simulink model "parallel_downconverter_test"  (Simulink 7.4)
settings: Solver=ode45  StartTime=0.0  StopTime=1000  RelTol=1e-3
undefined symbols (not defined in the file): Parallel_scope, Parallelizer, To_be_added_to_xBlocks_devels
libraries: xbsIndex_r4 x73, simulink x5
settings Model: Creator=chenhong  LastModifiedBy=hong

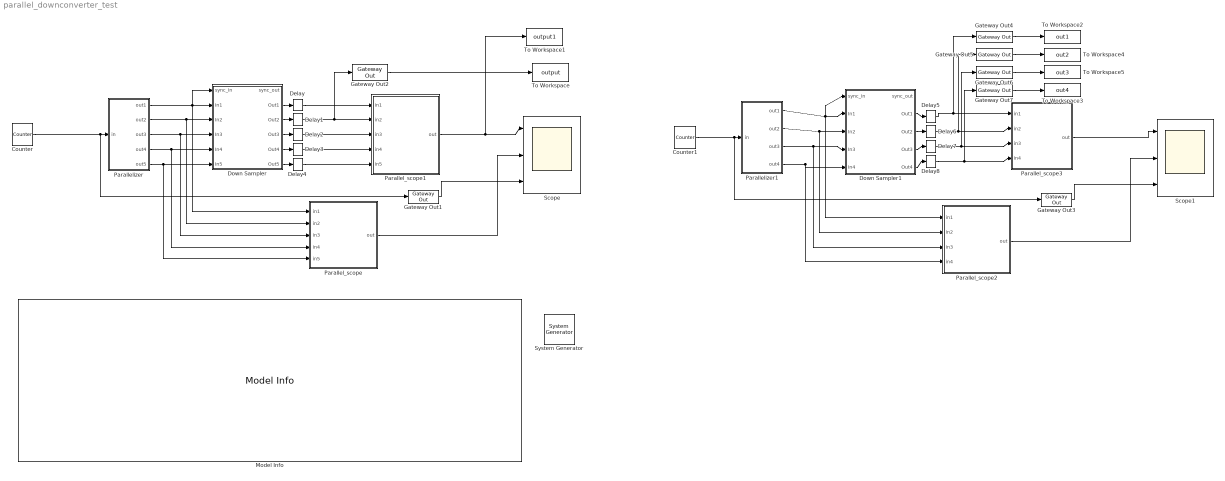
== system parallel_downconverter_test ==
  " System Generator" : xbsIndex_r4/ System Generator  Tag=genX  SystemSampleTime=-1  xilinxfamily=virtex6  part=xc6vsx315t  speed=-3  package=ff1156  synthesis_tool=XST  clock_wrapper=Clock Enables  directory=./netlist  testbench=off  simulink_period=1  sysclk_period=10  dcm_input_clock_period=10  incr_netlist=off  trim_vbits=Everywhere in SubSystem  dbl_ovrd=According to Block Masks  core_generation=According to Block Masks  run_coregen=off  deprecated_control=off  eval_field=0  block_type=sysgen
      settings: block_version=11.4
  Counter : xbsIndex_r4/Counter  cnt_type=Free Running  cnt_to=Inf  operation=Up  start_count=0  cnt_by_val=1  arith_type=Unsigned  n_bits=8  bin_pt=0  load_pin=off  rst=off  en=off  explicit_period=on  period=1  dbl_ovrd=off  use_behavioral_HDL=off  implementation=Fabric  block_type=counter
      settings: block_version=11.4
  Counter1 : xbsIndex_r4/Counter  cnt_type=Free Running  cnt_to=Inf  operation=Up  start_count=0  cnt_by_val=1  arith_type=Unsigned  n_bits=8  bin_pt=0  load_pin=off  rst=off  en=off  explicit_period=on  period=1  dbl_ovrd=off  use_behavioral_HDL=off  implementation=Fabric  block_type=counter
      settings: block_version=11.4
  Delay{,1..8} (9 alike) : xbsIndex_r4/Delay  en=off  latency=7  dbl_ovrd=off  reg_retiming=off  block_type=delay
      settings: block_version=11.4
  Down Sampler : Subsystem  mask(Parallel Downconverter (xBlock)){n_inputs=5, dec_rate=2, xilinx=off, input_clk_rate=5}
      mask prompts: n_inputs "number of inputs"; dec_rate "Decimation rate"; xilinx "Use Xilinx version of Down Sample?"; input_clk_rate "Input Clock Rate"
      mask help: Parallely downconvert.
      mask init:
      | config.source=str2func('parallel_downsampler_init_xblock');
      | config.depend=get_dependlist('parallel_downsampler');
      | config.toplevel=gcb;
      | set_param(gcb,'LinkStatus','inactive');
      | xBlock(config, {config.toplevel,...
      |     'n_inputs', n_inputs, ...
      |     'dec_rate', dec_rate, ...
      |     'xilinx', xilinx, ...
      |     'input_clk_rate', input_clk_rate});
      settings: AttributesFormatString=Decimation Rate = 2
  Down Sampler1 : Subsystem  mask(Parallel Downconverter (xBlock)){n_inputs=4, dec_rate=2, xilinx=off, input_clk_rate=4}
      mask prompts: n_inputs "number of inputs"; dec_rate "Decimation rate"; xilinx "Use Xilinx version of Down Sample?"; input_clk_rate "Input Clock Rate"
      mask help: Parallely downconvert.
      mask init: same as parallel_downconverter_test/Down Sampler
      settings: AttributesFormatString=Decimation Rate = 2
  Gateway Out{1..7} (7 alike) : xbsIndex_r4/Gateway Out  hdl_port=on  timing_constraint=None  locs_specified=off  LOCs={}  block_type=gatewayout
      settings: infoedit="Gateway out block.  Converts Xilinx fixed point inputs into ouputs of type Simulink integer, double, or fixed point.<br><br>Hardware notes:  In hardware these blocks become top level output ports or are discarded, depending on how they are configured."  block_version=11.4
  Model Info : simulink/Model-Wide Utilities/Model Info  SystemSampleTime=-1  InitialBlockCM=None  BlockCM=None  Frame=on  DisplayStringWithTags=|  HorizontalTextAlignment=Center  LeftAlignmentValue=0.5  SourceBlockDiagram=parallel_downconverter_test  TagMaxNumber=20
      | January 18, 2012:
      | 
      | Test passed.
      | 
      | Used downsample_init_xblock instead of the xilinx Down Sample block. Note that in this case it doesn't really change the sampling rate, just hold a certain value for a specific time. Therefore we need to adjust delays to see how they're matched.
      | 
      | To do: add option to choose the first value or last value in a single time frame.
      | 
      | 
      | ---------------------------------------------------------------
      | September 28, 2011:
      | 
      | Test passed. 
      | 
      | The counter generates 1-D discrete samples at 1 sample/clk rate. The parallelizer outputs 4-parallel outputs
      | at 4 sample/clk. The downconverter downsample to 4/dec_rate sample/clk. After the serializer, the final 1-D output stream is 1/dec_rate sample/clk.
      | 
      | 
      | Also tested: 5-parallel inputs; various dec_rate
  Parallel_scope : Subsystem  AncestorBlock=To_be_added_to_xBlocks_devels/Parallel_scope  mask(Parallel Scope){n_inputs=5, sample_period=5}
      mask prompts: n_inputs "Number of inputs"; sample_period "Sample Period"
      mask help:
      | This parallel scope can handle parallel inputs
      | by propagating though gateways and serialize into
      | one single stream. The output can then be connected
      | directly to a scope or toWorkspace.
      |
      | The sample_period desribes the parallel inputs rate.
      | For example, for a 4-inputs stream with sample_period = 1
      | (4 parallel inputs per Clk),  the output stream frequency
      | would be 4/1 = 4 (Sample/Clk)
      mask init:
      | config.source=str2func('parallel_scope_init_xblock');
      | config.depend=get_dependlist('parallel_scope');
      | config.toplevel=gcb;
      | set_param(gcb,'LinkStatus','inactive');
      | xBlock(config, {config.toplevel,...
      |     'n_inputs', n_inputs, ...
      |     'sample_period', sample_period});
      settings: AttributesFormatString=Sample Period = 5
  Parallel_scope1 : Subsystem  mask(Parallel Scope){n_inputs=5, sample_period=10, explicit_period=off}
      mask prompts: n_inputs "Number of inputs"; sample_period "Sample Period"; explicit_period "Explicit Period?"
      mask help:
      | This parallel scope can handle parallel inputs
      | by propagating though gateways and serialize into
      | one single stream. The output can then be connected
      | directly to a scope or toWorkspace.
      |
      | The sample_period desribes the parallel inputs rate.
      | For example, for a 4-inputs stream with sample_period = 1
      | (4 parallel inputs per Clk),  the output stream frequency
      | would be 4/1 = 4 (Sample/Clk)
      mask init:
      | config.source=str2func('parallel_scope_init_xblock');
      | config.depend=get_dependlist('parallel_scope');
      | config.toplevel=gcb;
      | set_param(gcb,'LinkStatus','inactive');
      | xBlock(config, {config.toplevel,...
      |     'n_inputs', n_inputs, ...
      |     'sample_period', sample_period, ...
      |     'explicit_period', explicit_period});
      settings: AttributesFormatString=Sample Period = 10
  Parallel_scope2 : Subsystem  AncestorBlock=To_be_added_to_xBlocks_devels/Parallel_scope  mask(Parallel Scope){n_inputs=4, sample_period=4}
      mask prompts: n_inputs "Number of inputs"; sample_period "Sample Period"
      mask help:
      | This parallel scope can handle parallel inputs
      | by propagating though gateways and serialize into
      | one single stream. The output can then be connected
      | directly to a scope or toWorkspace.
      |
      | The sample_period desribes the parallel inputs rate.
      | For example, for a 4-inputs stream with sample_period = 1
      | (4 parallel inputs per Clk),  the output stream frequency
      | would be 4/1 = 4 (Sample/Clk)
      mask init: same as parallel_downconverter_test/Parallel_scope
      settings: AttributesFormatString=Sample Period = 4
  Parallel_scope3 : Subsystem  mask(Parallel Scope){n_inputs=4, sample_period=8, explicit_period=off}
      mask prompts: n_inputs "Number of inputs"; sample_period "Sample Period"; explicit_period "Explicit Period?"
      mask help:
      | This parallel scope can handle parallel inputs
      | by propagating though gateways and serialize into
      | one single stream. The output can then be connected
      | directly to a scope or toWorkspace.
      |
      | The sample_period desribes the parallel inputs rate.
      | For example, for a 4-inputs stream with sample_period = 1
      | (4 parallel inputs per Clk),  the output stream frequency
      | would be 4/1 = 4 (Sample/Clk)
      mask init: same as parallel_downconverter_test/Parallel_scope1
      settings: AttributesFormatString=Sample Period = 8
  Parallelizer : Subsystem  AncestorBlock=To_be_added_to_xBlocks_devels/Parallelizer  mask(Parallelizer){n_outputs=5, sample_period=1}
      mask help:
      | Parallelizer takes in a single stream and convert it into
      | parallel outputs
      mask init:
      | config.source=str2func('parallelizer_init_xblock');
      | config.depend=get_dependlist('parallelizer');
      | config.toplevel=gcb;
      | set_param(gcb,'LinkStatus','inactive');
      | xBlock(config, {config.toplevel,...
      |     'n_outputs', n_outputs, ...
      |     'sample_period', sample_period});
      settings: AttributesFormatString=Sample Period = 1
  Parallelizer1 : Subsystem  AncestorBlock=To_be_added_to_xBlocks_devels/Parallelizer  mask(Parallelizer){n_outputs=4, sample_period=1}
      mask help:
      | Parallelizer takes in a single stream and convert it into
      | parallel outputs
      mask init: same as parallel_downconverter_test/Parallelizer
      settings: AttributesFormatString=Sample Period = 1
  Scope : Scope  NumInputPorts=3
      settings: YMin=-5~-5~-5  YMax=5~5~5
  Scope1 : Scope  NumInputPorts=3
      settings: YMin=-5~-5~-5  YMax=5~5~5
  To Workspace : ToWorkspace  VariableName=output  SampleTime=-1  SaveFormat=Structure
  To Workspace1 : ToWorkspace  VariableName=output1  SampleTime=-1  SaveFormat=Structure
  To Workspace2 : ToWorkspace  VariableName=out1  SampleTime=-1  SaveFormat=Structure
  To Workspace3 : ToWorkspace  VariableName=out4  SampleTime=-1  SaveFormat=Structure
  To Workspace4 : ToWorkspace  VariableName=out2  SampleTime=-1  SaveFormat=Structure
  To Workspace5 : ToWorkspace  VariableName=out3  SampleTime=-1  SaveFormat=Structure
  wires:
  Counter/1 -> Parallelizer/1(in), Gateway Out1/1
  Parallelizer/1(out1) -> Parallel_scope/1(in1), Down Sampler/1(sync_in), Down Sampler/2(In1)
  Parallelizer/2(out2) -> Parallel_scope/2(in2), Down Sampler/3(In2)
  Parallelizer/3(out3) -> Parallel_scope/3(in3), Down Sampler/4(In3)
  Parallelizer/4(out4) -> Parallel_scope/4(in4), Down Sampler/5(In4)
  Down Sampler/2(Out1) -> Delay/1
  Down Sampler/3(Out2) -> Delay1/1
  Down Sampler/4(Out3) -> Delay2/1
  Down Sampler/5(Out4) -> Delay3/1
  Parallel_scope1/1(out) -> Scope/1, To Workspace1/1
  Parallel_scope/1(out) -> Scope/2
  Gateway Out1/1 -> Scope/3
  Parallelizer/5(out5) -> Parallel_scope/5(in5), Down Sampler/6(In5)
  Down Sampler/6(Out5) -> Delay4/1
  Gateway Out2/1 -> To Workspace/1
  Delay/1 -> Parallel_scope1/1(in1)
  Delay1/1 -> Parallel_scope1/2(in2), Gateway Out2/1
  Delay2/1 -> Parallel_scope1/3(in3)
  Delay3/1 -> Parallel_scope1/4(in4)
  Delay4/1 -> Parallel_scope1/5(in5)
  Counter1/1 -> Parallelizer1/1(in), Gateway Out3/1
  Parallelizer1/1(out1) -> Parallel_scope2/1(in1), Down Sampler1/1(sync_in), Down Sampler1/2(In1)
  Parallelizer1/2(out2) -> Parallel_scope2/2(in2), Down Sampler1/3(In2)
  Parallelizer1/3(out3) -> Parallel_scope2/3(in3), Down Sampler1/4(In3)
  Parallelizer1/4(out4) -> Parallel_scope2/4(in4), Down Sampler1/5(In4)
  Down Sampler1/2(Out1) -> Delay5/1
  Down Sampler1/3(Out2) -> Delay6/1
  Down Sampler1/4(Out3) -> Delay7/1
  Down Sampler1/5(Out4) -> Delay8/1
  Parallel_scope3/1(out) -> Scope1/1
  Parallel_scope2/1(out) -> Scope1/2
  Gateway Out3/1 -> Scope1/3
  Delay5/1 -> Parallel_scope3/1(in1), Gateway Out4/1
  Delay6/1 -> Parallel_scope3/2(in2), Gateway Out5/1
  Delay7/1 -> Parallel_scope3/3(in3), Gateway Out6/1
  Delay8/1 -> Parallel_scope3/4(in4), Gateway Out7/1
  Gateway Out4/1 -> To Workspace2/1
  Gateway Out5/1 -> To Workspace4/1
  Gateway Out6/1 -> To Workspace5/1
  Gateway Out7/1 -> To Workspace3/1

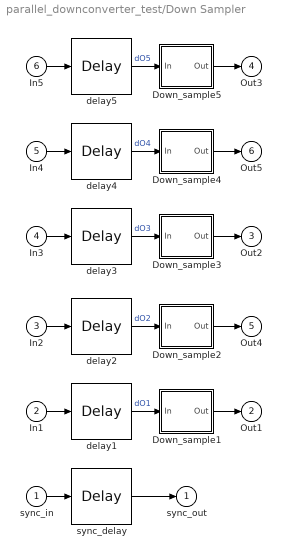
== system parallel_downconverter_test/Down Sampler ==
  sync_in : Inport
  In1 : Inport  Port=2
  In2 : Inport  Port=3
  In3 : Inport  Port=4
  In4 : Inport  Port=5
  In5 : Inport  Port=6
  Down_sample1 : Subsystem
  Down_sample2 : Subsystem
  Down_sample3 : Subsystem
  Down_sample4 : Subsystem
  Down_sample5 : Subsystem
  delay1 : xbsIndex_r4/Delay  en=off  latency=1  dbl_ovrd=off  reg_retiming=off  block_type=delay
      settings: block_version=11.4
  delay2 : xbsIndex_r4/Delay  en=off  latency=0  dbl_ovrd=off  reg_retiming=off  block_type=delay
      settings: block_version=11.4
  delay3 : xbsIndex_r4/Delay  en=off  latency=1  dbl_ovrd=off  reg_retiming=off  block_type=delay
      settings: block_version=11.4
  delay4 : xbsIndex_r4/Delay  en=off  latency=0  dbl_ovrd=off  reg_retiming=off  block_type=delay
      settings: block_version=11.4
  delay5 : xbsIndex_r4/Delay  en=off  latency=1  dbl_ovrd=off  reg_retiming=off  block_type=delay
      settings: block_version=11.4
  sync_delay : xbsIndex_r4/Delay  en=off  latency=1  dbl_ovrd=off  reg_retiming=off  block_type=delay
      settings: block_version=11.4
  sync_out : Outport
  Out1 : Outport  Port=2
  Out2 : Outport  Port=3
  Out3 : Outport  Port=4
  Out4 : Outport  Port=5
  Out5 : Outport  Port=6
  wires:
  sync_delay/1 -> sync_out/1
  sync_in/1 -> sync_delay/1
  Down_sample5/1(Out) -> Out3/1
  delay5/1 -> Down_sample5/1(In)  "dO5"
  In5/1 -> delay5/1
  Down_sample4/1(Out) -> Out5/1
  delay4/1 -> Down_sample4/1(In)  "dO4"
  In4/1 -> delay4/1
  Down_sample3/1(Out) -> Out2/1
  delay3/1 -> Down_sample3/1(In)  "dO3"
  In3/1 -> delay3/1
  Down_sample2/1(Out) -> Out4/1
  delay2/1 -> Down_sample2/1(In)  "dO2"
  In2/1 -> delay2/1
  Down_sample1/1(Out) -> Out1/1
  delay1/1 -> Down_sample1/1(In)  "dO1"
  In1/1 -> delay1/1

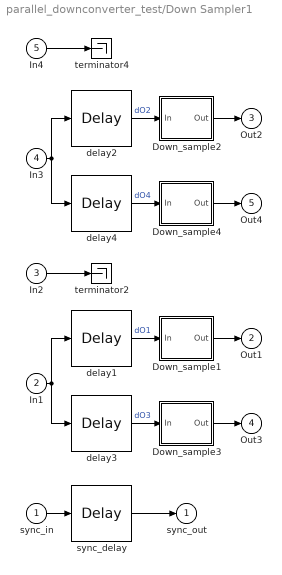
== system parallel_downconverter_test/Down Sampler1 ==
  sync_in : Inport
  In1 : Inport  Port=2
  In2 : Inport  Port=3
  In3 : Inport  Port=4
  In4 : Inport  Port=5
  Down_sample1 : Subsystem
  Down_sample2 : Subsystem
  Down_sample3 : Subsystem
  Down_sample4 : Subsystem
  delay1 : xbsIndex_r4/Delay  en=off  latency=1  dbl_ovrd=off  reg_retiming=off  block_type=delay
      settings: block_version=11.4
  delay2 : xbsIndex_r4/Delay  en=off  latency=1  dbl_ovrd=off  reg_retiming=off  block_type=delay
      settings: block_version=11.4
  delay3 : xbsIndex_r4/Delay  en=off  latency=0  dbl_ovrd=off  reg_retiming=off  block_type=delay
      settings: block_version=11.4
  delay4 : xbsIndex_r4/Delay  en=off  latency=0  dbl_ovrd=off  reg_retiming=off  block_type=delay
      settings: block_version=11.4
  sync_delay : xbsIndex_r4/Delay  en=off  latency=1  dbl_ovrd=off  reg_retiming=off  block_type=delay
      settings: block_version=11.4
  terminator2 : Terminator
  terminator4 : Terminator
  sync_out : Outport
  Out1 : Outport  Port=2
  Out2 : Outport  Port=3
  Out3 : Outport  Port=4
  Out4 : Outport  Port=5
  wires:
  In1/1 -> delay3/1, delay1/1
  In3/1 -> delay4/1, delay2/1
  sync_delay/1 -> sync_out/1
  sync_in/1 -> sync_delay/1
  Down_sample4/1(Out) -> Out4/1
  delay4/1 -> Down_sample4/1(In)  "dO4"
  Down_sample3/1(Out) -> Out3/1
  delay3/1 -> Down_sample3/1(In)  "dO3"
  Down_sample2/1(Out) -> Out2/1
  delay2/1 -> Down_sample2/1(In)  "dO2"
  Down_sample1/1(Out) -> Out1/1
  delay1/1 -> Down_sample1/1(In)  "dO1"
  In4/1 -> terminator4/1
  In2/1 -> terminator2/1

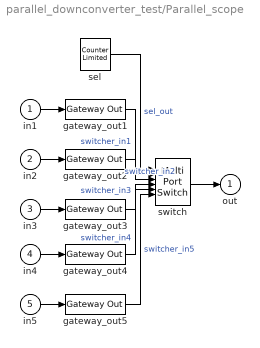
== system parallel_downconverter_test/Parallel_scope ==
  in1 : Inport
  in2 : Inport  Port=2
  in3 : Inport  Port=3
  in4 : Inport  Port=4
  in5 : Inport  Port=5
  gateway_out{1..5} (5 alike) : xbsIndex_r4/Gateway Out  hdl_port=off  timing_constraint=None  locs_specified=off  LOCs={}  block_type=gatewayout
      settings: infoedit="Gateway out block.  Converts Xilinx fixed point inputs into ouputs of type Simulink integer, double, or fixed point.<br><br>Hardware notes:  In hardware these blocks become top level output ports or are discarded, depending on how they are configured."  block_version=11.4
  sel : simulink/Sources/Counter Limited  SystemSampleTime=-1  uplimit=4  tsamp=1
  switch : MultiPortSwitch  Inputs=5  zeroidx=on  OutDataType=fixdt(1, 16)  OutScaling=2^0
  out : Outport
  wires:
  switch/1 -> out/1
  gateway_out5/1 -> switch/6  "switcher_in5"
  gateway_out4/1 -> switch/5  "switcher_in4"
  gateway_out3/1 -> switch/4  "switcher_in3"
  gateway_out2/1 -> switch/3  "switcher_in2"
  gateway_out1/1 -> switch/2  "switcher_in1"
  sel/1 -> switch/1  "sel_out"
  in5/1 -> gateway_out5/1
  in4/1 -> gateway_out4/1
  in3/1 -> gateway_out3/1
  in2/1 -> gateway_out2/1
  in1/1 -> gateway_out1/1

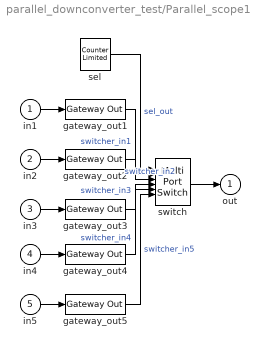
== system parallel_downconverter_test/Parallel_scope1 ==
  in1 : Inport
  in2 : Inport  Port=2
  in3 : Inport  Port=3
  in4 : Inport  Port=4
  in5 : Inport  Port=5
  gateway_out{1..5} (5 alike) : xbsIndex_r4/Gateway Out  hdl_port=off  timing_constraint=None  locs_specified=off  LOCs={}  block_type=gatewayout
      settings: infoedit="Gateway out block.  Converts Xilinx fixed point inputs into ouputs of type Simulink integer, double, or fixed point.<br><br>Hardware notes:  In hardware these blocks become top level output ports or are discarded, depending on how they are configured."  block_version=11.4
  sel : simulink/Sources/Counter Limited  SystemSampleTime=-1  uplimit=4  tsamp=2
  switch : MultiPortSwitch  Inputs=5  zeroidx=on  OutDataType=fixdt(1, 16)  OutScaling=2^0
  out : Outport
  wires:
  switch/1 -> out/1
  gateway_out5/1 -> switch/6  "switcher_in5"
  gateway_out4/1 -> switch/5  "switcher_in4"
  gateway_out3/1 -> switch/4  "switcher_in3"
  gateway_out2/1 -> switch/3  "switcher_in2"
  gateway_out1/1 -> switch/2  "switcher_in1"
  sel/1 -> switch/1  "sel_out"
  in5/1 -> gateway_out5/1
  in4/1 -> gateway_out4/1
  in3/1 -> gateway_out3/1
  in2/1 -> gateway_out2/1
  in1/1 -> gateway_out1/1

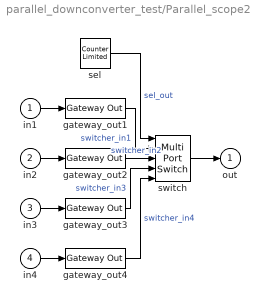
== system parallel_downconverter_test/Parallel_scope2 ==
  in1 : Inport
  in2 : Inport  Port=2
  in3 : Inport  Port=3
  in4 : Inport  Port=4
  gateway_out{1..4} (4 alike) : xbsIndex_r4/Gateway Out  hdl_port=off  timing_constraint=None  locs_specified=off  LOCs={}  block_type=gatewayout
      settings: infoedit="Gateway out block.  Converts Xilinx fixed point inputs into ouputs of type Simulink integer, double, or fixed point.<br><br>Hardware notes:  In hardware these blocks become top level output ports or are discarded, depending on how they are configured."  block_version=11.4
  sel : simulink/Sources/Counter Limited  SystemSampleTime=-1  uplimit=3  tsamp=1
  switch : MultiPortSwitch  Inputs=4  zeroidx=on  OutDataType=fixdt(1, 16)  OutScaling=2^0
  out : Outport
  wires:
  switch/1 -> out/1
  gateway_out4/1 -> switch/5  "switcher_in4"
  gateway_out3/1 -> switch/4  "switcher_in3"
  gateway_out2/1 -> switch/3  "switcher_in2"
  gateway_out1/1 -> switch/2  "switcher_in1"
  sel/1 -> switch/1  "sel_out"
  in4/1 -> gateway_out4/1
  in3/1 -> gateway_out3/1
  in2/1 -> gateway_out2/1
  in1/1 -> gateway_out1/1

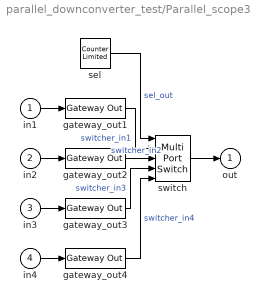
== system parallel_downconverter_test/Parallel_scope3 ==
  in1 : Inport
  in2 : Inport  Port=2
  in3 : Inport  Port=3
  in4 : Inport  Port=4
  gateway_out{1..4} (4 alike) : xbsIndex_r4/Gateway Out  hdl_port=off  timing_constraint=None  locs_specified=off  LOCs={}  block_type=gatewayout
      settings: infoedit="Gateway out block.  Converts Xilinx fixed point inputs into ouputs of type Simulink integer, double, or fixed point.<br><br>Hardware notes:  In hardware these blocks become top level output ports or are discarded, depending on how they are configured."  block_version=11.4
  sel : simulink/Sources/Counter Limited  SystemSampleTime=-1  uplimit=3  tsamp=2
  switch : MultiPortSwitch  Inputs=4  zeroidx=on  OutDataType=fixdt(1, 16)  OutScaling=2^0
  out : Outport
  wires:
  switch/1 -> out/1
  gateway_out4/1 -> switch/5  "switcher_in4"
  gateway_out3/1 -> switch/4  "switcher_in3"
  gateway_out2/1 -> switch/3  "switcher_in2"
  gateway_out1/1 -> switch/2  "switcher_in1"
  sel/1 -> switch/1  "sel_out"
  in4/1 -> gateway_out4/1
  in3/1 -> gateway_out3/1
  in2/1 -> gateway_out2/1
  in1/1 -> gateway_out1/1

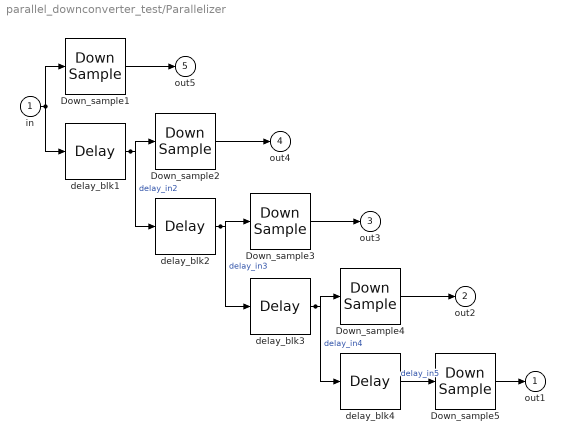
== system parallel_downconverter_test/Parallelizer ==
  in : Inport
  Down_sample{1..5} (5 alike) : xbsIndex_r4/Down Sample  sample_ratio=5  sample_phase="Last Value of Frame  (most efficient)"  en=off  latency=1  dbl_ovrd=off  block_type=dsamp
      settings: block_version=11.4
  delay_blk{1..4} (4 alike) : xbsIndex_r4/Delay  en=off  latency=1  dbl_ovrd=off  reg_retiming=off  block_type=delay
      settings: block_version=11.4
  out1 : Outport
  out2 : Outport  Port=2
  out3 : Outport  Port=3
  out4 : Outport  Port=4
  out5 : Outport  Port=5
  wires:
  in/1 -> Down_sample1/1, delay_blk1/1
  delay_blk1/1 -> Down_sample2/1, delay_blk2/1  "delay_in2"
  delay_blk2/1 -> Down_sample3/1, delay_blk3/1  "delay_in3"
  delay_blk3/1 -> Down_sample4/1, delay_blk4/1  "delay_in4"
  Down_sample5/1 -> out1/1
  delay_blk4/1 -> Down_sample5/1  "delay_in5"
  Down_sample4/1 -> out2/1
  Down_sample3/1 -> out3/1
  Down_sample2/1 -> out4/1
  Down_sample1/1 -> out5/1

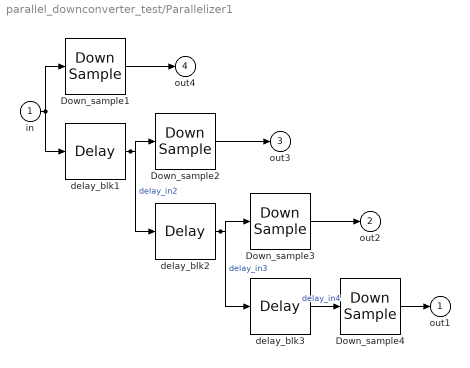
== system parallel_downconverter_test/Parallelizer1 ==
  in : Inport
  Down_sample{1..4} (4 alike) : xbsIndex_r4/Down Sample  sample_ratio=4  sample_phase="Last Value of Frame  (most efficient)"  en=off  latency=1  dbl_ovrd=off  block_type=dsamp
      settings: block_version=11.4
  delay_blk1 : xbsIndex_r4/Delay  en=off  latency=1  dbl_ovrd=off  reg_retiming=off  block_type=delay
      settings: block_version=11.4
  delay_blk2 : xbsIndex_r4/Delay  en=off  latency=1  dbl_ovrd=off  reg_retiming=off  block_type=delay
      settings: block_version=11.4
  delay_blk3 : xbsIndex_r4/Delay  en=off  latency=1  dbl_ovrd=off  reg_retiming=off  block_type=delay
      settings: block_version=11.4
  out1 : Outport
  out2 : Outport  Port=2
  out3 : Outport  Port=3
  out4 : Outport  Port=4
  wires:
  in/1 -> Down_sample1/1, delay_blk1/1
  delay_blk1/1 -> Down_sample2/1, delay_blk2/1  "delay_in2"
  delay_blk2/1 -> Down_sample3/1, delay_blk3/1  "delay_in3"
  Down_sample4/1 -> out1/1
  delay_blk3/1 -> Down_sample4/1  "delay_in4"
  Down_sample3/1 -> out2/1
  Down_sample2/1 -> out3/1
  Down_sample1/1 -> out4/1

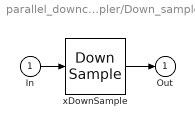
== system parallel_downconverter_test/Down Sampler/Down_sample1 ==
  In : Inport
  xDownSample : xbsIndex_r4/Down Sample  sample_ratio=2  sample_phase="Last Value of Frame  (most efficient)"  en=off  latency=1  dbl_ovrd=off  block_type=dsamp
      settings: block_version=11.4
  Out : Outport
  wires:
  xDownSample/1 -> Out/1
  In/1 -> xDownSample/1

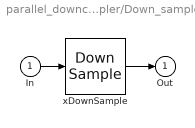
== system parallel_downconverter_test/Down Sampler/Down_sample2 ==
  In : Inport
  xDownSample : xbsIndex_r4/Down Sample  sample_ratio=2  sample_phase="Last Value of Frame  (most efficient)"  en=off  latency=1  dbl_ovrd=off  block_type=dsamp
      settings: block_version=11.4
  Out : Outport
  wires:
  xDownSample/1 -> Out/1
  In/1 -> xDownSample/1

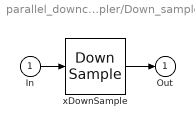
== system parallel_downconverter_test/Down Sampler/Down_sample3 ==
  In : Inport
  xDownSample : xbsIndex_r4/Down Sample  sample_ratio=2  sample_phase="Last Value of Frame  (most efficient)"  en=off  latency=1  dbl_ovrd=off  block_type=dsamp
      settings: block_version=11.4
  Out : Outport
  wires:
  xDownSample/1 -> Out/1
  In/1 -> xDownSample/1

== system parallel_downconverter_test/Down Sampler/Down_sample4 ==
  In : Inport
  xDownSample : xbsIndex_r4/Down Sample  sample_ratio=2  sample_phase="Last Value of Frame  (most efficient)"  en=off  latency=1  dbl_ovrd=off  block_type=dsamp
      settings: block_version=11.4
  Out : Outport
  wires:
  xDownSample/1 -> Out/1
  In/1 -> xDownSample/1

== system parallel_downconverter_test/Down Sampler/Down_sample5 ==
  In : Inport
  xDownSample : xbsIndex_r4/Down Sample  sample_ratio=2  sample_phase="Last Value of Frame  (most efficient)"  en=off  latency=1  dbl_ovrd=off  block_type=dsamp
      settings: block_version=11.4
  Out : Outport
  wires:
  xDownSample/1 -> Out/1
  In/1 -> xDownSample/1

== system parallel_downconverter_test/Down Sampler1/Down_sample1 ==
  In : Inport
  xDownSample : xbsIndex_r4/Down Sample  sample_ratio=2  sample_phase="Last Value of Frame  (most efficient)"  en=off  latency=1  dbl_ovrd=off  block_type=dsamp
      settings: block_version=11.4
  Out : Outport
  wires:
  xDownSample/1 -> Out/1
  In/1 -> xDownSample/1

== system parallel_downconverter_test/Down Sampler1/Down_sample2 ==
  In : Inport
  xDownSample : xbsIndex_r4/Down Sample  sample_ratio=2  sample_phase="Last Value of Frame  (most efficient)"  en=off  latency=1  dbl_ovrd=off  block_type=dsamp
      settings: block_version=11.4
  Out : Outport
  wires:
  xDownSample/1 -> Out/1
  In/1 -> xDownSample/1

== system parallel_downconverter_test/Down Sampler1/Down_sample3 ==
  In : Inport
  xDownSample : xbsIndex_r4/Down Sample  sample_ratio=2  sample_phase="Last Value of Frame  (most efficient)"  en=off  latency=1  dbl_ovrd=off  block_type=dsamp
      settings: block_version=11.4
  Out : Outport
  wires:
  xDownSample/1 -> Out/1
  In/1 -> xDownSample/1

== system parallel_downconverter_test/Down Sampler1/Down_sample4 ==
  In : Inport
  xDownSample : xbsIndex_r4/Down Sample  sample_ratio=2  sample_phase="Last Value of Frame  (most efficient)"  en=off  latency=1  dbl_ovrd=off  block_type=dsamp
      settings: block_version=11.4
  Out : Outport
  wires:
  xDownSample/1 -> Out/1
  In/1 -> xDownSample/1
